simulink model "speed_control_SPWM_Five_phase_PMSM"  (R2015a)
settings: Solver=ode3  StartTime=0.0  StopTime=0.2  FixedStep=0.0000001  MaxStep=0.000001  MinStep=0.0000001  RelTol=1e-3
libraries: powerlib x19, simulink x5, powerlib_meascontrol x2
settings Model: Creator=hp  LastModifiedBy=hp

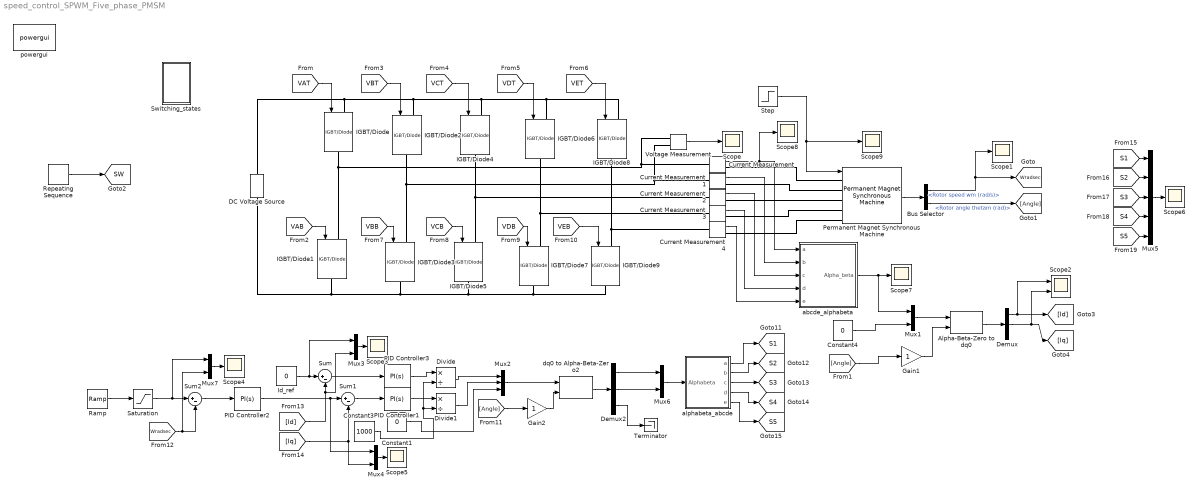
== system speed_control_SPWM_Five_phase_PMSM ==
  Alpha-Beta-Zero to dq0 : powerlib_meascontrol/Transformations/Alpha-Beta-Zero to dq0  Alignment=Aligned with phase A axis
  Bus Selector : BusSelector  OutputSignals=Rotor speed wm (rad/s),Rotor angle thetam (rad)
  Constant1 : Constant  Value=0
  Constant3 : Constant  Value=1000
  Constant4 : Constant  Value=0
  Current Measurement{,1..4} (5 alike) : powerlib/Measurements/Current Measurement  PhasorSimulation=off  OutputType=Complex  PSBequivalent=0
  DC Voltage Source : powerlib/Electrical Sources/DC Voltage Source  Amplitude=1000  Measurements=None
  Demux : Demux  Outputs=3
  Demux2 : Demux  Outputs=3
  Divide : Product  Inputs=*/
  Divide1 : Product  Inputs=*/
  Gain1 : Gain
  Gain2 : Gain
  IGBT/Diode{,1..9} (10 alike) : powerlib/Power Electronics/IGBT//Diode  Ron=1e-3  Rs=1e5  Cs=inf  Measurements=off
  Id_ref : Constant  Value=0
  Mux{1,3..4,6..7} (5 alike) : Mux  Inputs=2
  Mux2 : Mux  Inputs=3
  Mux5 : Mux  Inputs=5
  PID Controller1 : simulink/Continuous/PID Controller  Controller=PI  TimeDomain=Continuous-time  SampleTime=-1  IntegratorMethod=Forward Euler  FilterMethod=Forward Euler  Form=Parallel  UseFilter=on  ControllerParametersSource=internal  P=40  I=15000  D=0  N=100  InitialConditionSource=internal  InitialConditionForIntegrator=0  InitialConditionForFilter=0  ExternalReset=none  LimitOutput=off  UpperSaturationLimit=inf  LowerSaturationLimit=-inf  LinearizeAsGain=on  AntiWindupMode=none  Kb=1  TrackingMode=off  Kt=1  PParamMin=[]  PParamMax=[]  IParamMin=[]  IParamMax=[]  DParamMin=[]  DParamMax=[]  NParamMin=[]  NParamMax=[]  KbParamMin=[]  KbParamMax=[]  KtParamMin=[]  KtParamMax=[]  POutMin=[]  POutMax=[]  IOutMin=[]  IOutMax=[]  DOutMin=[]  DOutMax=[]  NOutMin=[]  NOutMax=[]  KbOutMin=[]  KbOutMax=[]  KtOutMin=[]  KtOutMax=[]  IntegratorOutMin=[]  IntegratorOutMax=[]  FilterOutMin=[]  FilterOutMax=[]  SumOutMin=[]  SumOutMax=[]  SumI1OutMin=[]  SumI1OutMax=[]  SumI2OutMin=[]  SumI2OutMax=[]  SumI3OutMin=[]  SumI3OutMax=[]  SumDOutMin=[]  SumDOutMax=[]  SaturationOutMin=[]  SaturationOutMax=[]  IntegratorContinuousStateAttributes=''  IntegratorStateMustResolveToSignalObject=off  IntegratorRTWStateStorageClass=Auto  FilterContinuousStateAttributes=''  FilterStateMustResolveToSignalObject=off  FilterRTWStateStorageClass=Auto  DifferentiatorICPrevScaledInput=0  DifferentiatorOutMin=[]  DifferentiatorOutMax=[]
  PID Controller2 : simulink/Continuous/PID Controller  Controller=PI  TimeDomain=Continuous-time  SampleTime=-1  IntegratorMethod=Forward Euler  FilterMethod=Forward Euler  Form=Parallel  UseFilter=on  ControllerParametersSource=internal  P=60  I=10000  D=0  N=100  InitialConditionSource=internal  InitialConditionForIntegrator=0  InitialConditionForFilter=0  ExternalReset=none  LimitOutput=off  UpperSaturationLimit=inf  LowerSaturationLimit=-inf  LinearizeAsGain=on  AntiWindupMode=none  Kb=1  TrackingMode=off  Kt=1  PParamMin=[]  PParamMax=[]  IParamMin=[]  IParamMax=[]  DParamMin=[]  DParamMax=[]  NParamMin=[]  NParamMax=[]  KbParamMin=[]  KbParamMax=[]  KtParamMin=[]  KtParamMax=[]  POutMin=[]  POutMax=[]  IOutMin=[]  IOutMax=[]  DOutMin=[]  DOutMax=[]  NOutMin=[]  NOutMax=[]  KbOutMin=[]  KbOutMax=[]  KtOutMin=[]  KtOutMax=[]  IntegratorOutMin=[]  IntegratorOutMax=[]  FilterOutMin=[]  FilterOutMax=[]  SumOutMin=[]  SumOutMax=[]  SumI1OutMin=[]  SumI1OutMax=[]  SumI2OutMin=[]  SumI2OutMax=[]  SumI3OutMin=[]  SumI3OutMax=[]  SumDOutMin=[]  SumDOutMax=[]  SaturationOutMin=[]  SaturationOutMax=[]  IntegratorContinuousStateAttributes=''  IntegratorStateMustResolveToSignalObject=off  IntegratorRTWStateStorageClass=Auto  FilterContinuousStateAttributes=''  FilterStateMustResolveToSignalObject=off  FilterRTWStateStorageClass=Auto  DifferentiatorICPrevScaledInput=0  DifferentiatorOutMin=[]  DifferentiatorOutMax=[]
  PID Controller3 : simulink/Continuous/PID Controller  Controller=PI  TimeDomain=Continuous-time  SampleTime=-1  IntegratorMethod=Forward Euler  FilterMethod=Forward Euler  Form=Parallel  UseFilter=on  ControllerParametersSource=internal  P=40  I=15000  D=0  N=100  InitialConditionSource=internal  InitialConditionForIntegrator=0  InitialConditionForFilter=0  ExternalReset=none  LimitOutput=off  UpperSaturationLimit=inf  LowerSaturationLimit=-inf  LinearizeAsGain=on  AntiWindupMode=none  Kb=1  TrackingMode=off  Kt=1  PParamMin=[]  PParamMax=[]  IParamMin=[]  IParamMax=[]  DParamMin=[]  DParamMax=[]  NParamMin=[]  NParamMax=[]  KbParamMin=[]  KbParamMax=[]  KtParamMin=[]  KtParamMax=[]  POutMin=[]  POutMax=[]  IOutMin=[]  IOutMax=[]  DOutMin=[]  DOutMax=[]  NOutMin=[]  NOutMax=[]  KbOutMin=[]  KbOutMax=[]  KtOutMin=[]  KtOutMax=[]  IntegratorOutMin=[]  IntegratorOutMax=[]  FilterOutMin=[]  FilterOutMax=[]  SumOutMin=[]  SumOutMax=[]  SumI1OutMin=[]  SumI1OutMax=[]  SumI2OutMin=[]  SumI2OutMax=[]  SumI3OutMin=[]  SumI3OutMax=[]  SumDOutMin=[]  SumDOutMax=[]  SaturationOutMin=[]  SaturationOutMax=[]  IntegratorContinuousStateAttributes=''  IntegratorStateMustResolveToSignalObject=off  IntegratorRTWStateStorageClass=Auto  FilterContinuousStateAttributes=''  FilterStateMustResolveToSignalObject=off  FilterRTWStateStorageClass=Auto  DifferentiatorICPrevScaledInput=0  DifferentiatorOutMin=[]  DifferentiatorOutMax=[]
  Permanent Magnet Synchronous Machine : powerlib/Machines/Permanent Magnet Synchronous Machine  NbPhases=5  FluxDistribution=Sinusoidal  RotorType=Round  MechanicalLoad=Torque Tm  PresetModel=No  ShowDetailedParameters=on  MeasurementBus=off  Resistance=2.0  Inductance=8.5e-3  dqInductances=[8.5e-3,8.5e-3]  La=0.005  MachineConstant=Flux linkage established by magnets (V.s)  Flux=0.1194  VoltageCst=14.6988  TorqueCst=0.2985  Flat=120  Mechanical=[0.0027 0.0004924 1 0]  PolePairs=4  InitialConditions=[0,0, 0,0]  InitialConditions5ph=[0 0 0 0 0 0]  TsPowergui=0  TsBlock=-1  RefAngle=Aligned with phase A axis (original Park)
  Ramp : simulink/Sources/Ramp  slope=10000  start=0  X0=0
  Repeating Sequence : simulink/Sources/Repeating Sequence  rep_seq_t=[0 0.25 0.5 0.75 1.0]/10000  rep_seq_y=[0 1 0 -1 0]
  Saturation : Saturate  UpperLimit=300  LowerLimit=-300
  Scope{,1,3..9} (9 alike) : Scope
      Scope settings: YMin=-100  YMax=110
      Scope1 settings: YMin=-9e-14  YMax=1.26218e-29  SaveName=ScopeData9
      Scope3 settings: TimeRange=0.2  YMin=-0.0075  YMax=0.025  SaveName=ScopeData10
      Scope4 settings: TimeRange=0.2  YMin=-10  YMax=400  SaveName=ScopeData13
      Scope5 settings: YMin=-16.31  YMax=-16.23  SaveName=ScopeData11
      Scope6 settings: YMin=-0.275  YMax=0.25  SaveName=ScopeData6
      Scope7 settings: YMin=-17.5  YMax=17.5  SaveName=ScopeData7
      Scope8 settings: YMin=-35  YMax=35  SaveName=ScopeData8
      Scope9 settings: YMin=-0.275  YMax=0.25  SaveName=ScopeData14
  Scope2 : Scope  NumInputPorts=2
      settings: YMin=9.89~-2e-15  YMax=10.1~7.5e-15  SaveName=ScopeData12
  Step : Step  Time=0.1  Before=10  After=-5  SampleTime=0
  Sum : Sum  Inputs=|+-
  Sum1 : Sum  Inputs=|+-
  Sum2 : Sum  Inputs=|+-
  Switching_states : Subsystem
  Terminator : Terminator
  Voltage Measurement : powerlib/Measurements/Voltage Measurement  PhasorSimulation=off  OutputType=Complex  PSBequivalent=0
  abcde_alphabeta : Subsystem
  alphabeta_abcde : Subsystem
  dq0 to Alpha-Beta-Zero2 : powerlib_meascontrol/Transformations/dq0 to Alpha-Beta-Zero  Alignment=Aligned with phase A axis
  powergui : powerlib/powergui  Priority=1  SimulationMode=Continuous  SolverType=Tustin/Backward Euler (TBE)  SampleTime=50e-6  frequency=60  SPID=off  DisableSnubberDevices=off  DisableRonSwitches=off  DisableVfSwitches=off  SwTol=0  DisplayEquations=off  Interpol=off  methode=off  Ts=100  FunctionMessages=off  echomessages=off  HookPort=off  EnableUseOfTLC=off  x0status=blocks  frequencyindice=0  Pbase=100e6  ErrMax=1e-4  Iterations=50  UnitsV=kV  UnitsW=MW  buscounter=0  RestoreLinks=warning  ResistiveCurrentMeasurement=off  Frange=[0:2:500]  Ylog=off  Xlog=on  ShowGrid=off  save=off  variable=ZData  structure=ScopeData  ZoomFFT=off  StartTime=0.0  cycles=10  DisplayStyle=1  fundamental=50  FreqAxis=off  MaxFrequency=1000  frequencyindicesteady=1  RmsSteady=1  display=off
  tag scope: S1=global, S2=global, S3=global, S4=global, S5=global, SW=global, Wradsec=global
  wires:
  [VAT] -> IGBT/Diode/1
  Repeating Sequence/1 -> [SW]
  [VAB] -> IGBT/Diode1/1
  [VBT] -> IGBT/Diode2/1
  [VCT] -> IGBT/Diode4/1
  [VDT] -> IGBT/Diode6/1
  [VET] -> IGBT/Diode8/1
  [VBB] -> IGBT/Diode3/1
  [VCB] -> IGBT/Diode5/1
  [VDB] -> IGBT/Diode7/1
  [VEB] -> IGBT/Diode9/1
  Voltage Measurement/1 -> Scope/1
  [S1] -> Mux5/1
  [S2] -> Mux5/2
  [S3] -> Mux5/3
  [S4] -> Mux5/4
  [S5] -> Mux5/5
  Mux5/1 -> Scope6/1
  Current Measurement4/1 -> abcde_alphabeta/5(e)
  Current Measurement3/1 -> abcde_alphabeta/4(d)
  Current Measurement2/1 -> abcde_alphabeta/3(c)
  Current Measurement1/1 -> abcde_alphabeta/2(b)
  Current Measurement/1 -> Scope8/1, abcde_alphabeta/1(a)
  abcde_alphabeta/1(Alpha_beta) -> Mux1/1, Scope7/1
  Permanent Magnet Synchronous Machine/1 -> Bus Selector/1
  Step/1 -> Scope9/1, Permanent Magnet Synchronous Machine/1
  Bus Selector/1 -> Scope1/1, [Wradsec]  "<Rotor speed wm (rad/s)>"
  Constant4/1 -> Mux1/2
  Alpha-Beta-Zero to dq0/1 -> Demux/1
  Mux1/1 -> Alpha-Beta-Zero to dq0/1
  Demux/1 -> Scope2/1, [Id]
  Demux/2 -> Scope2/2, [Iq]
  dq0 to Alpha-Beta-Zero2/1 -> Demux2/1
  Demux2/2 -> Mux6/2
  Demux2/3 -> Terminator/1
  [Angle] -> Gain2/1
  Gain2/1 -> dq0 to Alpha-Beta-Zero2/2
  Mux2/1 -> dq0 to Alpha-Beta-Zero2/1
  Sum/1 -> PID Controller3/1
  Sum1/1 -> PID Controller1/1
  Mux3/1 -> Scope3/1
  [Iq] -> Mux4/2, Sum1/2
  Mux4/1 -> Scope5/1
  [Id] -> Mux3/2, Sum/2
  PID Controller1/1 -> Divide1/1
  PID Controller3/1 -> Divide/1
  Divide/1 -> Mux2/1
  Divide1/1 -> Mux2/2
  Constant1/1 -> Mux2/3
  Constant3/1 -> Divide/2, Divide1/2
  PID Controller2/1 -> Mux4/1, Sum1/1
  Id_ref/1 -> Mux3/1, Sum/1
  Mux6/1 -> alphabeta_abcde/1(Alphabeta)
  Demux2/1 -> Mux6/1
  alphabeta_abcde/3(c) -> [S3]
  alphabeta_abcde/1(a) -> [S1]
  alphabeta_abcde/2(b) -> [S2]
  alphabeta_abcde/4(d) -> [S4]
  alphabeta_abcde/5(e) -> [S5]
  [Angle] -> Gain1/1
  Gain1/1 -> Alpha-Beta-Zero to dq0/2
  Bus Selector/2 -> [Angle]  "<Rotor angle thetam (rad)>"
  Sum2/1 -> PID Controller2/1
  Saturation/1 -> Mux7/1, Sum2/1
  Ramp/1 -> Saturation/1
  Mux7/1 -> Scope4/1
  [Wradsec] -> Sum2/2, Mux7/2
  connections:
  IGBT/Diode/RConn1 -- Current Measurement/LConn1 -- Voltage Measurement/LConn1 -- IGBT/Diode1/LConn1
  IGBT/Diode3/LConn1 -- Current Measurement1/LConn1 -- Voltage Measurement/LConn2 -- IGBT/Diode2/RConn1
  IGBT/Diode5/LConn1 -- Current Measurement2/LConn1 -- IGBT/Diode4/RConn1
  IGBT/Diode7/LConn1 -- Current Measurement3/LConn1 -- IGBT/Diode6/RConn1
  IGBT/Diode9/LConn1 -- Current Measurement4/LConn1 -- IGBT/Diode8/RConn1
  DC Voltage Source/LConn1 -- IGBT/Diode1/RConn1 -- IGBT/Diode3/RConn1 -- IGBT/Diode5/RConn1 -- IGBT/Diode7/RConn1 -- IGBT/Diode9/RConn1
  IGBT/Diode8/LConn1 -- IGBT/Diode6/LConn1 -- IGBT/Diode4/LConn1 -- IGBT/Diode2/LConn1 -- IGBT/Diode/LConn1 -- DC Voltage Source/RConn1
  Permanent Magnet Synchronous Machine/LConn1 -- Current Measurement/RConn1
  Permanent Magnet Synchronous Machine/LConn2 -- Current Measurement1/RConn1
  Current Measurement2/RConn1 -- Permanent Magnet Synchronous Machine/LConn3
  Permanent Magnet Synchronous Machine/LConn4 -- Current Measurement3/RConn1
  Current Measurement4/RConn1 -- Permanent Magnet Synchronous Machine/LConn5

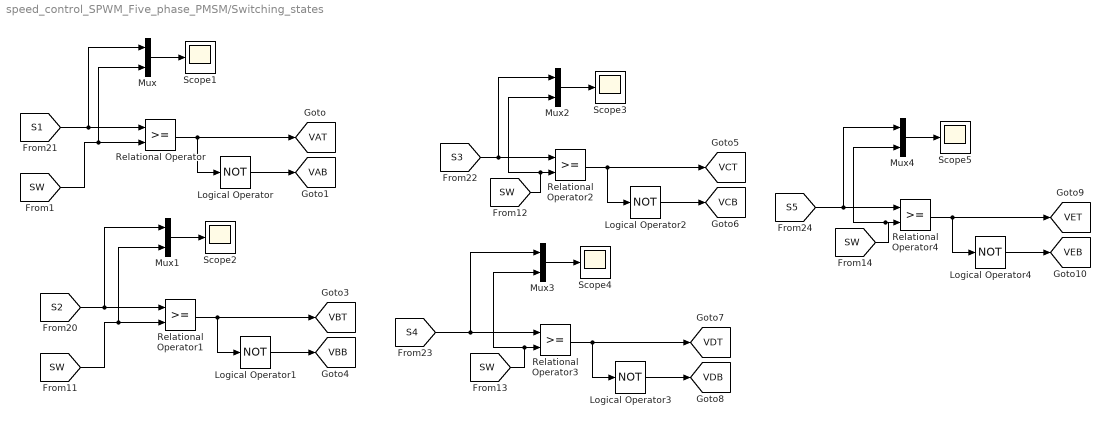
== system speed_control_SPWM_Five_phase_PMSM/Switching_states ==
  Logical Operator{,1..4} (5 alike) : Logic  Operator=NOT  Inputs=1  AllPortsSameDT=off  OutDataTypeStr=boolean
  Mux{,1..4} (5 alike) : Mux  Inputs=2
  Relational Operator{,1..4} (5 alike) : RelationalOperator  OutDataTypeStr=boolean
  Scope{1..5} (5 alike) : Scope
      Scope1 settings: YMin=-1  YMax=1
      Scope2 settings: YMin=-1  YMax=1  SaveName=ScopeData2
      Scope3 settings: YMin=-1  YMax=1  SaveName=ScopeData3
      Scope4 settings: YMin=-1  YMax=1  SaveName=ScopeData4
      Scope5 settings: YMin=-1  YMax=1  SaveName=ScopeData5
  tag scope: VAB=global, VAT=global, VBB=global, VBT=global, VCB=global, VCT=global, VDB=global, VDT=global, VEB=global, VET=global
  wires:
  [S5] -> Mux4/1, Relational Operator4/1
  [S3] -> Mux2/1, Relational Operator2/1
  [S4] -> Mux3/1, Relational Operator3/1
  [S2] -> Mux1/1, Relational Operator1/1
  [S1] -> Mux/1, Relational Operator/1
  Logical Operator/1 -> [VAB]
  Relational Operator/1 -> Logical Operator/1, [VAT]
  [SW] -> Mux/2, Relational Operator/2
  Mux/1 -> Scope1/1
  [SW] -> Mux1/2, Relational Operator1/2
  Relational Operator4/1 -> Logical Operator4/1, [VET]
  Logical Operator2/1 -> [VCB]
  [SW] -> Mux2/2, Relational Operator2/2
  [SW] -> Mux4/2, Relational Operator4/2
  Logical Operator1/1 -> [VBB]
  Logical Operator3/1 -> [VDB]
  Mux1/1 -> Scope2/1
  Mux2/1 -> Scope3/1
  Mux4/1 -> Scope5/1
  Relational Operator2/1 -> Logical Operator2/1, [VCT]
  Mux3/1 -> Scope4/1
  [SW] -> Mux3/2, Relational Operator3/2
  Logical Operator4/1 -> [VEB]
  Relational Operator1/1 -> Logical Operator1/1, [VBT]
  Relational Operator3/1 -> Logical Operator3/1, [VDT]

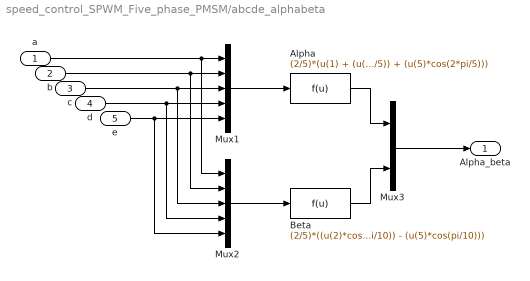
== system speed_control_SPWM_Five_phase_PMSM/abcde_alphabeta ==
  a : Inport
  b : Inport  Port=2
  c : Inport  Port=3
  d : Inport  Port=4
  e : Inport  Port=5
  Alpha : Fcn  Expr=(2/5)*(u(1) + (u(2)*cos(2*pi/5)) + (u(3)*cos(4*pi/5)) + (u(4)*cos(4*pi/5)) + (u(5)*cos(2*pi/5)))
  Beta : Fcn  Expr=(2/5)*((u(2)*cos(pi/10)) + (u(3)*cos(3*pi/10)) - (u(4)*cos(3*pi/10)) - (u(5)*cos(pi/10)))
  Mux1 : Mux  Inputs=5
  Mux2 : Mux  Inputs=5
  Mux3 : Mux  Inputs=2
  Alpha_beta : Outport
  wires:
  Mux1/1 -> Alpha/1
  Beta/1 -> Mux3/2
  Mux2/1 -> Beta/1
  Alpha/1 -> Mux3/1
  Mux3/1 -> Alpha_beta/1
  a/1 -> Mux2/1, Mux1/1
  b/1 -> Mux2/2, Mux1/2
  c/1 -> Mux2/3, Mux1/3
  d/1 -> Mux2/4, Mux1/4
  e/1 -> Mux2/5, Mux1/5

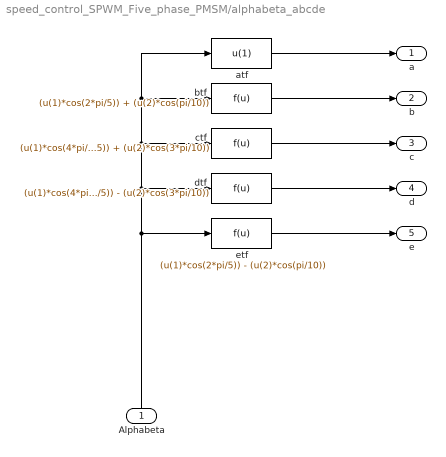
== system speed_control_SPWM_Five_phase_PMSM/alphabeta_abcde ==
  Alphabeta : Inport
  atf : Fcn  Expr=u(1)
  btf : Fcn  Expr=(u(1)*cos(2*pi/5)) + (u(2)*cos(pi/10))
  ctf : Fcn  Expr=(u(1)*cos(4*pi/5)) + (u(2)*cos(3*pi/10))
  dtf : Fcn  Expr=(u(1)*cos(4*pi/5)) - (u(2)*cos(3*pi/10))
  etf : Fcn  Expr=(u(1)*cos(2*pi/5)) - (u(2)*cos(pi/10))
  a : Outport
  b : Outport  Port=2
  c : Outport  Port=3
  d : Outport  Port=4
  e : Outport  Port=5
  wires:
  atf/1 -> a/1
  btf/1 -> b/1
  dtf/1 -> d/1
  etf/1 -> e/1
  ctf/1 -> c/1
  Alphabeta/1 -> etf/1, ctf/1, atf/1, btf/1, dtf/1
